simulink model "rb_openloop"  (R2019a)
settings: Solver=VariableStepAuto  StartTime=0.0  StopTime=10.0  RelTol=1e-3
undefined symbols (not defined in the file): Ion, Lithium
libraries: powerlib x10, powerlib_meascontrol x7, electricdrivelib x1
settings Model: Creator=ishan  LastModifiedBy=ishan

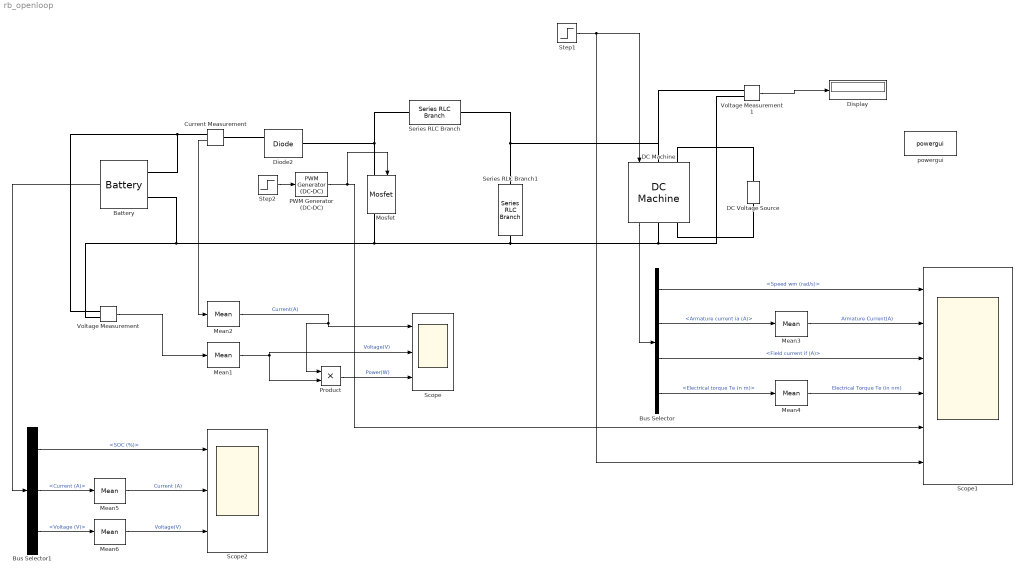
== system rb_openloop ==
  Battery : electricdrivelib/Extra Sources/Battery  BatType=Lithium-Ion  ShowTempParam=off  ThermalPreset=no  ShowAgeParam=off  NomV=240  NomQ=20  SOC=50  Batt_Tr=30  PresetModel=on  MaxQ=20  MinV=180  FullV=279.3569  Dis_rate=8.6957  R=0.12  Normal_OP=18.087  expZone="[259.2926     0.9826087]"  current=[6.5 13 32.5]  Units=Time  Tci=20  NomT=20  T2=-30  MaxQ2=4.8  FullV2=7.1  Normal_OP2=5.655  expZone2="[6.58           1]"  Rca=0.6  ti=2000  Dp=0  Neq0=0  Tsim=1e6  Ta1=25  Qeol=5.4*0.9  Reol=0.013333*1.2  Char_age=[2.3478, 3]  Dis_age=[2.3478, 10]  N1=1500  N2=10500  N3=1000  N4=1400  Ta2=45  N5=950
      settings: SourceProductName=Simscape Electrical
  Bus Selector : BusSelector  OutputSignals=Speed wm (rad/s),Armature current ia (A),Field current if (A),Electrical torque Te (n m)
  Bus Selector1 : BusSelector  OutputSignals=SOC (%),Current (A),Voltage (V)
  Current Measurement : powerlib/Measurements/Current Measurement  PhasorSimulation=off  OutputType=Complex  PSBequivalent=0
      settings: SourceProductName=Simscape Electrical
  DC Machine : powerlib/Machines/DC Machine  PresetModel=01: 5HP 240V 1750RPM Field:300V  MechanicalLoad=Torque TL  FieldType=Wound  ShowDetailedParameters=on  MeasurementBus=off  RLa=[2.581 0.028]  RLf=[281.3 156]  Laf=0.9483  MachineConstant=Torque constant (N.m/A)  Ke=1.8  Kt=1.8  J=0.02215  Bm=0.002953  Tf=0.5161  w0=1  Ifinit=1  TsPowergui=0  TsBlock=-1
      settings: SourceProductName=Simscape Electrical
  DC Voltage Source : powerlib/Electrical Sources/DC Voltage Source  Amplitude=300  Measurements=None
      settings: SourceProductName=Simscape Electrical
  Diode2 : powerlib/Power Electronics/Diode  Ron=0.001  Lon=0  Vf=0.8  IC=0  UseSnubber=0  Rs=500  Cs=250e-9  Measurements=on
      settings: SourceProductName=Simscape Electrical
  Display : Display
  Mean{1..6} (6 alike) : powerlib_meascontrol/Measurements/Mean  Freq=60  Vinit=0  Ts=0
      settings: SourceProductName=Simscape Electrical
  Mosfet : powerlib/Power Electronics/Mosfet  Ron=0.1  Lon=0  Rd=0.01  Vfd=0  IC=0  Rs=1e5  Cs=inf  Measurements=on
      settings: SourceProductName=Simscape Electrical
  PWM Generator (DC-DC) : powerlib_meascontrol/Pulse & Signal Generators/PWM Generator (DC-DC)  Fsw=5000  Ts=0
      settings: SourceProductName=Simscape Electrical
  Product : Product
  Scope : Scope  NumInputPorts=3
  Scope1 : Scope  NumInputPorts=6
  Scope2 : Scope  NumInputPorts=3
  Series RLC Branch : powerlib/Elements/Series RLC Branch  LConnTagsString=__new0  RConnTagsString=__new0  BranchType=L  Resistance=1  Inductance=5e-3  SetiL0=off  InitialCurrent=0  Capacitance=1e-6  Setx0=off  InitialVoltage=0  Measurements=None
      settings: SourceProductName=Simscape Electrical
  Series RLC Branch1 : powerlib/Elements/Series RLC Branch  LConnTagsString=__new0  RConnTagsString=__new0  BranchType=C  Resistance=1  Inductance=1e-3  SetiL0=off  InitialCurrent=0  Capacitance=150e-6  Setx0=off  InitialVoltage=0  Measurements=None
      settings: SourceProductName=Simscape Electrical
  Step1 : Step  Time=5  Before=-20  After=-15  SampleTime=0
  Step2 : Step  Time=3  Before=0.6  After=0.8  SampleTime=0
  Voltage Measurement : powerlib/Measurements/Voltage Measurement  PhasorSimulation=off  OutputType=Complex  PSBequivalent=0
      settings: SourceProductName=Simscape Electrical
  Voltage Measurement1 : powerlib/Measurements/Voltage Measurement  PhasorSimulation=off  OutputType=Magnitude  PSBequivalent=0
      settings: SourceProductName=Simscape Electrical
  powergui : powerlib/powergui  Priority=1  SimulationMode=Continuous  SampleTime=50e-6  frequency=60  Iterations=50  frequencyindice=0  Pbase=100e6  ErrMax=1e-4  UnitsV=kV  UnitsW=MW  buscounter=0  FunctionMessages=off  echomessages=off  EnableUseOfTLC=off  CurrentSourceSwitches=off  DisableSnubberDevices=off  DisableRonSwitches=off  DisableVfSwitches=off  DisplayEquations=off  AutomaticDiscreteSolvers=off  SolverType=Tustin/Backward Euler (TBE)  Interpol=off  ExternalGateDelay=off  methode=off  Ts=100  x0status=blocks  SPID=on  SwTol=0  HookPort=off  NonlinearTolerance=0  nMaxIteration=15  ContinueOnMaxIteration=off  RestoreLinks=warning  ResistiveCurrentMeasurement=off  Frange=[0:2:500]  Ylog=off  Xlog=on  ShowGrid=off  save=off  variable=ZData  structure=0  ZoomFFT=off  StartTime=0.0  cycles=1  DisplayStyle=1  fundamental=60  FreqAxis=off  MaxFrequency=1000  frequencyindicesteady=1  RmsSteady=1  display=off
      settings: SourceProductName=Simscape Electrical
  wires:
  Voltage Measurement/1 -> Mean1/1
  Mean1/1 -> Scope/2, Product/2  "Voltage(V)"
  Mean2/1 -> Product/1, Scope/1  "Current(A)"
  Product/1 -> Scope/3  "Power(W)"
  DC Machine/1 -> Bus Selector/1
  Bus Selector/2 -> Mean3/1  "<Armature current ia (A)>"
  Bus Selector/1 -> Scope1/1  "<Speed wm (rad/s)>"
  Bus Selector/3 -> Scope1/3  "<Field current if (A)>"
  Bus Selector/4 -> Mean4/1  "<Electrical torque Te (n m)>"
  Current Measurement/1 -> Mean2/1
  Battery/1 -> Bus Selector1/1
  Bus Selector1/2 -> Mean5/1  "<Current (A)>"
  Bus Selector1/1 -> Scope2/1  "<SOC (%)>"
  Bus Selector1/3 -> Mean6/1  "<Voltage (V)>"
  Voltage Measurement1/1 -> Display/1
  Step1/1 -> Scope1/6, DC Machine/1
  Mean3/1 -> Scope1/2  "Armature Current(A)"
  Mean4/1 -> Scope1/4  "Electrical Torque Te (in nm)"
  Mean5/1 -> Scope2/2  "Current (A)"
  Step2/1 -> PWM Generator (DC-DC)/1
  PWM Generator (DC-DC)/1 -> Scope1/5, Mosfet/1
  Mean6/1 -> Scope2/3  "Voltage(V)"
  connections:
  Series RLC Branch/RConn1 -- Voltage Measurement1/LConn1 -- DC Machine/LConn1 -- Series RLC Branch1/LConn1
  Mosfet/LConn1 -- Diode2/LConn1 -- Series RLC Branch/LConn1
  DC Machine/LConn2 -- DC Voltage Source/RConn1
  DC Machine/RConn2 -- DC Voltage Source/LConn1
  DC Machine/RConn1 -- Voltage Measurement1/LConn2 -- Series RLC Branch1/RConn1 -- Mosfet/RConn1 -- Voltage Measurement/LConn2 -- Battery/LConn2
  Battery/LConn1 -- Voltage Measurement/LConn1 -- Current Measurement/RConn1
  Current Measurement/LConn1 -- Diode2/RConn1
